simulink model "Mat_func_1"  (R2015b)
settings: Solver=VariableStepAuto  StartTime=0.0  StopTime=8000  RelTol=1e-3
settings Model: Creator=asuS  LastModifiedBy=asuS

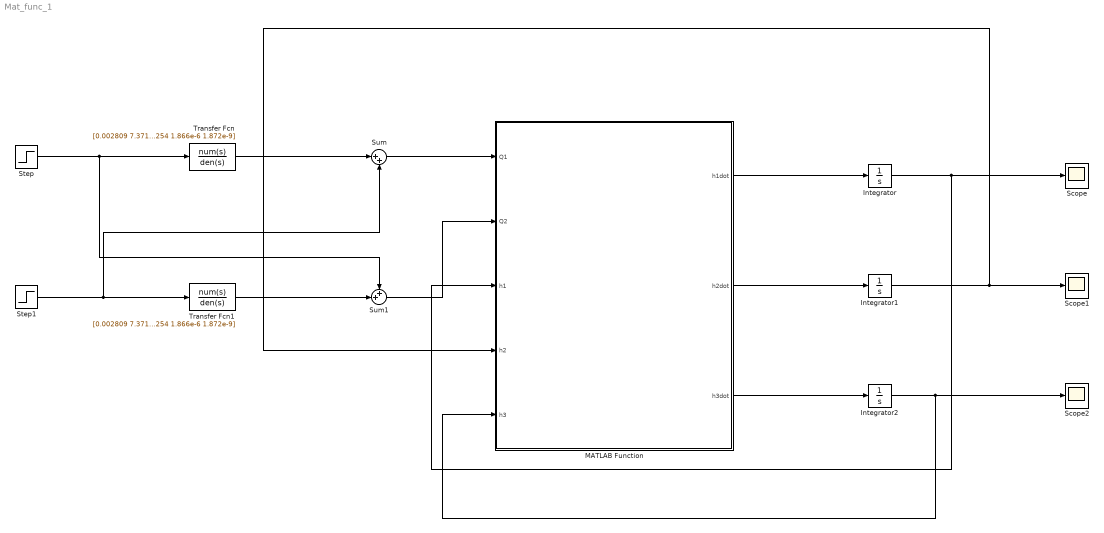
== system Mat_func_1 ==
  Integrator : Integrator
  Integrator1 : Integrator
  Integrator2 : Integrator
  MATLAB Function : MATLAB Function  TreatAsAtomicUnit=on
  Scope : Scope
  Scope1 : Scope
  Scope2 : Scope
  Step : Step  Time=0  After=3.4899e-5  SampleTime=0
  Step1 : Step  Time=0  After=3.4899e-5  SampleTime=0
  Sum : Sum  Inputs=|++
  Sum1 : Sum  Inputs=++|
  Transfer Fcn : TransferFcn  Numerator=[0.002809 7.371e-5 4.264e-7 6.056e-10]  Denominator=[64.65 4.261 0.08461 0.0006254 1.866e-6 1.872e-9]
  Transfer Fcn1 : TransferFcn  Numerator=[0.002809 7.371e-5 4.264e-7 6.056e-10]  Denominator=[64.65 4.261 0.08461 0.0006254 1.866e-6 1.872e-9]
  wires:
  MATLAB Function/3(h3dot) -> Integrator2/1
  MATLAB Function/2(h2dot) -> Integrator1/1
  MATLAB Function/1(h1dot) -> Integrator/1
  Integrator/1 -> MATLAB Function/3(h1), Scope/1
  Integrator1/1 -> MATLAB Function/4(h2), Scope1/1
  Integrator2/1 -> MATLAB Function/5(h3), Scope2/1
  Step/1 -> Sum1/1, Transfer Fcn/1
  Transfer Fcn/1 -> Sum/1
  Sum/1 -> MATLAB Function/1(Q1)
  Step1/1 -> Sum/2, Transfer Fcn1/1
  Transfer Fcn1/1 -> Sum1/2
  Sum1/1 -> MATLAB Function/2(Q2)

== matlab function Mat_func_1/MATLAB Function ==
  data: Q1 input; h1dot output; Q2 input; h1 input; h2 input; h3 input; h2dot output; h3dot output
function [h1dot, h2dot, h3dot] = fcn(Q1,Q2,h1,h2,h3)

h1dot = 64.935*(Q1) - 7.216*10^(-3)*sqrt(abs(h1 - h2));
h2dot = 7.216*10^(-3)*(sqrt(abs(h1 - h2)) + sqrt(abs(h3 - h2))) - 0.0101 *sqrt(abs(h2));
h3dot = 64.935*(Q2) - 7.216*10^(-3)*sqrt(abs(h3 - h2));

end
